simulink model "open loop simulationHbridgeMLI"  (R2019a)
settings: Solver=VariableStepAuto  StartTime=0.0  StopTime=0.2  RelTol=1e-3
libraries: powerlib x73, simulink x13, powerlib_meascontrol x3
settings Model: Creator=BPW  LastModifiedBy=BPW

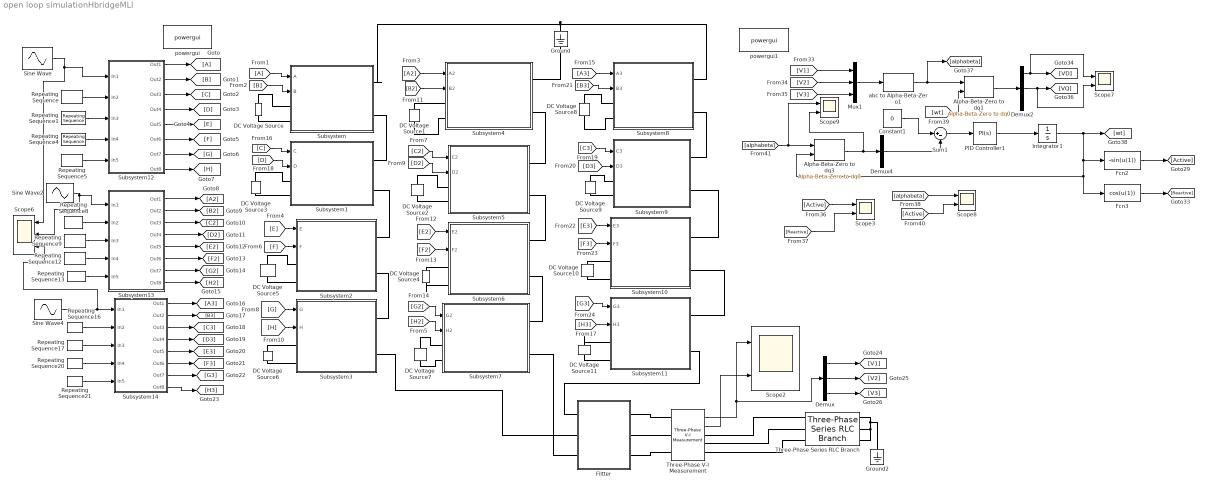
== system open loop simulationHbridgeMLI ==
  Alpha-Beta-Zero to dq1 : powerlib_meascontrol/Transformations/Alpha-Beta-Zero to dq0  Alignment=90 degrees behind phase A axis
      settings: SourceProductName=Simscape Electrical
  Alpha-Beta-Zero to dq3 : powerlib_meascontrol/Transformations/Alpha-Beta-Zero to dq0  Alignment=90 degrees behind phase A axis
      settings: SourceProductName=Simscape Electrical
  Constant1 : Constant  Value=0
  DC Voltage Source{,1..11} (12 alike) : powerlib/Electrical Sources/DC Voltage Source  Amplitude=-100  Measurements=None
      settings: SourceProductName=Simscape Electrical
  Demux : Demux  Outputs=3
  Demux2 : Demux  Outputs=3
  Demux4 : Demux  Outputs=3
  Fcn2 : Fcn  Expr=-sin(u(1))
  Fcn3 : Fcn  Expr=cos(u(1))
  Filtter : Subsystem
  Ground : powerlib/Elements/Ground  LConnTagsString=a
      settings: SourceProductName=Simscape Electrical
  Ground2 : powerlib/Elements/Ground  LConnTagsString=a
      settings: SourceProductName=Simscape Electrical
  Integrator1 : Integrator
  Mux1 : Mux  Inputs=3
  PID Controller1 : simulink/Continuous/PID Controller  Controller=PI  Form=Parallel  TimeDomain=Continuous-time  SampleTime=-1  IntegratorMethod=Forward Euler  FilterMethod=Forward Euler  ControllerParametersSource=internal  P=1  I=170  D=0  UseFilter=on  N=100  TunerSelectOption=Transfer Function Based (PID Tuner App)  InitialConditionSource=internal  InitialConditionForIntegrator=0  InitialConditionForFilter=0  DifferentiatorICPrevScaledInput=0  ExternalReset=none  TrackingMode=off  Kt=1  LimitOutput=off  UpperSaturationLimit=inf  LowerSaturationLimit=-inf  LinearizeAsGain=on  AntiWindupMode=none  Kb=1  POutMin=[]  POutMax=[]  IOutMin=[]  IOutMax=[]  DOutMin=[]  DOutMax=[]  NOutMin=[]  NOutMax=[]  SumOutMin=[]  SumOutMax=[]  SaturationOutMin=[]  SaturationOutMax=[]  PParamMin=[]  PParamMax=[]  IParamMin=[]  IParamMax=[]  DParamMin=[]  DParamMax=[]  NParamMin=[]  NParamMax=[]  KbParamMin=[]  KbParamMax=[]  KtParamMin=[]  KtParamMax=[]  KbOutMin=[]  KbOutMax=[]  KtOutMin=[]  KtOutMax=[]  IntegratorOutMin=[]  IntegratorOutMax=[]  FilterOutMin=[]  FilterOutMax=[]  SumI1OutMin=[]  SumI1OutMax=[]  SumI2OutMin=[]  SumI2OutMax=[]  SumI3OutMin=[]  SumI3OutMax=[]  SumI4OutMin=[]  SumI4OutMax=[]  SumDOutMin=[]  SumDOutMax=[]  DifferentiatorOutMin=[]  DifferentiatorOutMax=[]  FilterDiffOutCoefMin=[]  FilterDiffOutCoefMax=[]  ReciprocalOutMin=[]  ReciprocalOutMax=[]  SumDenOutMin=[]  SumDenOutMax=[]  SumNumOutMin=[]  SumNumOutMax=[]  DivideOutMin=[]  DivideOutMax=[]  IntegratorContinuousStateAttributes=''  IntegratorStateMustResolveToSignalObject=off  IntegratorRTWStateStorageClass=Auto  FilterContinuousStateAttributes=''  FilterStateMustResolveToSignalObject=off  FilterRTWStateStorageClass=Auto  ParallelPVariant=InternalParameters  IdealPVariant=Disabled  IVariant=InternalParameters  DVariant=Disabled  IntegratorVariant=Continuous  SatVariant=Disabled  AWVariant=Passthrough  PCopyVariant=Disabled  TRVariant=Disabled  FdbkBlocksVariant=Forward  IdealPFdbkVariant=Disabled  SatFdbkVariant=Disabled  DerivativeFilterVariant=Disabled  NVariant=Disabled  NCopyVariant=Disabled_SignalSpec  FilterICVariant=Disabled  IntegratorICVariant=InternalICs  ExternalResetVariant=Disabled  TRSumVariant=Passthrough  SumFdbkVariant=Disabled  SumVariant=Sum_PI
  Repeating Sequence : simulink/Sources/Repeating Sequence  rep_seq_t=[0 1e-4]  rep_seq_y=[0 1]
  Repeating Sequence1 : simulink/Sources/Repeating Sequence  rep_seq_t=[0 1e-4]  rep_seq_y=[1 2]
  Repeating Sequence12 : simulink/Sources/Repeating Sequence  rep_seq_t=[0 1e-4]  rep_seq_y=[2 3]
  Repeating Sequence13 : simulink/Sources/Repeating Sequence  rep_seq_t=[0 1e-4]  rep_seq_y=[3 4]
  Repeating Sequence16 : simulink/Sources/Repeating Sequence  rep_seq_t=[0 1e-4]  rep_seq_y=[0 1]
  Repeating Sequence17 : simulink/Sources/Repeating Sequence  rep_seq_t=[0 1e-4]  rep_seq_y=[1 2]
  Repeating Sequence20 : simulink/Sources/Repeating Sequence  rep_seq_t=[0 1e-4]  rep_seq_y=[2 3]
  Repeating Sequence21 : simulink/Sources/Repeating Sequence  rep_seq_t=[0 1e-4]  rep_seq_y=[3 4]
  Repeating Sequence4 : simulink/Sources/Repeating Sequence  rep_seq_t=[0 1e-4]  rep_seq_y=[2 3]
  Repeating Sequence5 : simulink/Sources/Repeating Sequence  rep_seq_t=[0 1e-4]  rep_seq_y=[3 4]
  Repeating Sequence8 : simulink/Sources/Repeating Sequence  rep_seq_t=[0 1e-4]  rep_seq_y=[0 1]
  Repeating Sequence9 : simulink/Sources/Repeating Sequence  rep_seq_t=[0 1e-4]  rep_seq_y=[1 2]
  Scope{2..3,7..9} (5 alike) : Scope  NumInputPorts=2
  Scope6 : Scope  NumInputPorts=3
  Sine Wave : Sin  Amplitude=4  Frequency=314.15  SampleTime=0
  Sine Wave2 : Sin  Amplitude=4  Frequency=314.15  Phase=2*pi/3  SampleTime=0
  Sine Wave4 : Sin  Amplitude=4  Frequency=314.15  Phase=4*pi/3  SampleTime=0
  Subsystem : Subsystem
  Subsystem1 : Subsystem
  Subsystem10 : Subsystem
  Subsystem11 : Subsystem
  Subsystem12 : Subsystem
  Subsystem13 : Subsystem
  Subsystem14 : Subsystem
  Subsystem2 : Subsystem
  Subsystem3 : Subsystem
  Subsystem4 : Subsystem
  Subsystem5 : Subsystem
  Subsystem6 : Subsystem
  Subsystem7 : Subsystem
  Subsystem8 : Subsystem
  Subsystem9 : Subsystem
  Sum1 : Sum  Inputs=|+-
  Three-Phase Series RLC Branch : powerlib/Elements/Three-Phase Series RLC Branch  LConnTagsString=A|B|C  RConnTagsString=A|B|C  BranchType=R  Resistance=10  Inductance=1e-9  Capacitance=1e-6  Measurements=None
      settings: SourceProductName=Simscape Electrical
  Three-Phase V-I Measurement : powerlib/Measurements/Three-Phase V-I Measurement  VoltageMeasurement=phase-to-ground  SetLabelV=off  LabelV=Vabc  Vpu=off  VpuLL=off  CurrentMeasurement=yes  SetLabelI=off  LabelI=Iabc  Ipu=off  Pbase=100e6  Vbase=500e3  OutputType=Complex  PhasorSimulation=off  PSBequivalent=0
      settings: SourceProductName=Simscape Electrical
  abc to Alpha-Beta-Zero1 : powerlib_meascontrol/Transformations/abc to Alpha-Beta-Zero
      settings: SourceProductName=Simscape Electrical
  powergui : powerlib/powergui  Priority=1  SimulationMode=Discrete  SampleTime=5e-5  frequency=60  Iterations=50  frequencyindice=0  Pbase=100e6  ErrMax=1e-4  UnitsV=kV  UnitsW=MW  buscounter=0  FunctionMessages=off  echomessages=off  EnableUseOfTLC=off  CurrentSourceSwitches=off  DisableSnubberDevices=off  DisableRonSwitches=off  DisableVfSwitches=off  DisplayEquations=off  AutomaticDiscreteSolvers=off  SolverType=Tustin/Backward Euler (TBE)  Interpol=off  ExternalGateDelay=off  methode=off  Ts=100  x0status=blocks  SPID=on  SwTol=0  HookPort=off  NonlinearTolerance=0  nMaxIteration=15  ContinueOnMaxIteration=off  RestoreLinks=warning  ResistiveCurrentMeasurement=off  Frange=[0:2:500]  Ylog=off  Xlog=on  ShowGrid=off  save=off  variable=ZData  structure=0  ZoomFFT=off  StartTime=0.0  cycles=1  DisplayStyle=1  fundamental=60  FreqAxis=off  MaxFrequency=1000  frequencyindicesteady=1  RmsSteady=1  display=off
      settings: SourceProductName=Simscape Electrical
  powergui1 : powerlib/powergui  Priority=1  SimulationMode=Discrete  SampleTime=5e-5  frequency=60  Iterations=50  frequencyindice=0  Pbase=100e6  ErrMax=1e-4  UnitsV=kV  UnitsW=MW  buscounter=0  FunctionMessages=off  echomessages=off  EnableUseOfTLC=off  CurrentSourceSwitches=off  DisableSnubberDevices=off  DisableRonSwitches=off  DisableVfSwitches=off  DisplayEquations=off  AutomaticDiscreteSolvers=off  SolverType=Tustin/Backward Euler (TBE)  Interpol=off  ExternalGateDelay=off  methode=off  Ts=100  x0status=blocks  SPID=on  SwTol=0  HookPort=off  NonlinearTolerance=0  nMaxIteration=15  ContinueOnMaxIteration=off  RestoreLinks=warning  ResistiveCurrentMeasurement=off  Frange=[0:2:500]  Ylog=off  Xlog=on  ShowGrid=off  save=off  variable=ZData  structure=0  ZoomFFT=off  StartTime=0.0  cycles=1  DisplayStyle=1  fundamental=60  FreqAxis=off  MaxFrequency=1000  frequencyindicesteady=1  RmsSteady=1  display=off
      settings: SourceProductName=Simscape Electrical
  wires:
  [B3] -> Subsystem8/2("B3 ")
  [A3] -> Subsystem8/1(A3)
  [F3] -> Subsystem10/2(F3)
  [C3] -> Subsystem9/1("C3 ")
  [E3] -> Subsystem10/1(E3)
  [H2] -> Subsystem7/2("H2 ")
  [B2] -> Subsystem4/2("B2 ")
  [G2] -> Subsystem7/1(G2)
  [C] -> Subsystem1/1(C)
  [H3] -> Subsystem11/2("H3 ")
  [E2] -> Subsystem6/1(E2)
  [F] -> Subsystem2/2(F)
  [A] -> Subsystem/1(A)
  [C2] -> Subsystem5/1(C2)
  [F2] -> Subsystem6/2(F2)
  [D] -> Subsystem1/2("D ")
  [D3] -> Subsystem9/2("D3 ")
  [B] -> Subsystem/2(B)
  [H] -> Subsystem3/2("H ")
  [G] -> Subsystem3/1(G)
  [A2] -> Subsystem4/1("A2 ")
  [G3] -> Subsystem11/1(G3)
  [E] -> Subsystem2/1(E)
  [D2] -> Subsystem5/2("D2 ")
  Three-Phase V-I Measurement/2 -> Scope2/2
  Demux/1 -> [V1]
  Demux/3 -> [V3]
  Demux/2 -> [V2]
  Three-Phase V-I Measurement/1 -> Scope2/1, Demux/1
  Subsystem12/7(Out7) -> [G]
  Subsystem12/4(Out4) -> [D]
  Subsystem12/6(Out6) -> [F]
  Subsystem14/3(Out3) -> [C3]
  Repeating Sequence20/1 -> Subsystem14/4(In4)
  Subsystem14/6(Out6) -> [F3]
  Subsystem12/2(Out2) -> [B]
  Repeating Sequence/1 -> Subsystem12/2(In2)
  Repeating Sequence1/1 -> Subsystem12/3(In3)
  Subsystem12/3(Out3) -> [C]
  Subsystem12/8(Out8) -> [H]
  Subsystem12/5(Out5) -> [E]
  Subsystem13/7(Out7) -> [G2]
  Subsystem13/6(Out6) -> [F2]
  Subsystem13/8(Out8) -> [H2]
  Subsystem12/1(Out1) -> [A]
  Subsystem13/4(Out4) -> [D2]
  Subsystem13/2(Out2) -> [B2]
  Subsystem13/1(Out1) -> [A2]
  Subsystem14/7(Out7) -> [G3]
  Repeating Sequence21/1 -> Subsystem14/5(In5)
  Repeating Sequence5/1 -> Subsystem12/5(In5)
  Repeating Sequence8/1 -> Subsystem13/2(In2)
  Subsystem14/8(Out8) -> [H3]
  Repeating Sequence17/1 -> Subsystem14/3(In3)
  Sine Wave2/1 -> Scope6/2, Subsystem13/1(In1)
  Repeating Sequence13/1 -> Subsystem13/5(In5)
  Repeating Sequence16/1 -> Subsystem14/2(In2)
  Subsystem14/1(Out1) -> [A3]
  Subsystem14/2(Out2) -> [B3]
  Sine Wave4/1 -> Scope6/3, Subsystem14/1(In1)
  Subsystem14/4(Out4) -> [D3]
  Subsystem13/5(Out5) -> [E2]
  Subsystem14/5(Out5) -> [E3]
  Repeating Sequence4/1 -> Subsystem12/4(In4)
  Sine Wave/1 -> Scope6/1, Subsystem12/1(In1)
  Subsystem13/3(Out3) -> [C2]
  Repeating Sequence12/1 -> Subsystem13/4(In4)
  Repeating Sequence9/1 -> Subsystem13/3(In3)
  [alphabeta] -> Scope8/1
  Demux4/2 -> Sum1/2
  Demux2/1 -> [VD], Scope7/1
  Alpha-Beta-Zero to dq1/1 -> Demux2/1
  Fcn3/1 -> [Reactive]
  [Active] -> Scope3/1
  Integrator1/1 -> Fcn2/1, Fcn3/1, Alpha-Beta-Zero to dq3/2, [wt]
  Demux2/2 -> Scope7/2, [VQ]
  [Reactive] -> Scope3/2
  [Active] -> Scope8/2
  Fcn2/1 -> [Active]
  Mux1/1 -> abc to Alpha-Beta-Zero1/1
  [V1] -> Mux1/1
  [wt] -> Alpha-Beta-Zero to dq1/2
  abc to Alpha-Beta-Zero1/1 -> Alpha-Beta-Zero to dq1/1, [alphabeta]
  Constant1/1 -> Sum1/1
  [V3] -> Mux1/3
  [alphabeta] -> Scope9/1, Alpha-Beta-Zero to dq3/1
  PID Controller1/1 -> Integrator1/1
  Alpha-Beta-Zero to dq3/1 -> Scope9/2, Demux4/1
  Sum1/1 -> PID Controller1/1
  [V2] -> Mux1/2
  connections:
  Ground/LConn1 -- Subsystem/RConn1 -- Subsystem4/RConn1 -- Subsystem8/RConn1
  Subsystem3/LConn1 -- DC Voltage Source6/RConn1
  Subsystem8/LConn1 -- DC Voltage Source8/RConn1
  Subsystem8/LConn2 -- DC Voltage Source8/LConn1
  Subsystem11/LConn2 -- DC Voltage Source11/LConn1
  Subsystem2/LConn1 -- DC Voltage Source5/RConn1
  Subsystem2/LConn2 -- DC Voltage Source5/LConn1
  Subsystem10/RConn2 -- Subsystem11/RConn1
  Subsystem10/RConn1 -- Subsystem9/RConn2
  Subsystem10/LConn1 -- DC Voltage Source10/RConn1
  Subsystem4/LConn1 -- DC Voltage Source1/RConn1
  Subsystem5/LConn2 -- DC Voltage Source2/LConn1
  Subsystem2/RConn1 -- Subsystem1/RConn2
  Subsystem5/LConn1 -- DC Voltage Source2/RConn1
  Subsystem7/LConn2 -- DC Voltage Source7/LConn1
  Subsystem6/RConn1 -- Subsystem5/RConn2
  Subsystem4/RConn2 -- Subsystem5/RConn1
  Subsystem6/LConn1 -- DC Voltage Source4/RConn1
  Subsystem8/RConn2 -- Subsystem9/RConn1
  Subsystem9/LConn1 -- DC Voltage Source9/RConn1
  Subsystem2/RConn2 -- Subsystem3/RConn1
  Subsystem9/LConn2 -- DC Voltage Source9/LConn1
  Subsystem3/LConn2 -- DC Voltage Source6/LConn1
  Subsystem4/LConn2 -- DC Voltage Source1/LConn1
  Subsystem6/RConn2 -- Subsystem7/RConn1
  Subsystem/RConn2 -- Subsystem1/RConn1
  Subsystem10/LConn2 -- DC Voltage Source10/LConn1
  Subsystem/LConn2 -- DC Voltage Source/LConn1
  Subsystem1/LConn1 -- DC Voltage Source3/RConn1
  Three-Phase Series RLC Branch/LConn1 -- Ground2/LConn1 -- Three-Phase Series RLC Branch/LConn3 -- Three-Phase Series RLC Branch/LConn2
  Three-Phase Series RLC Branch/RConn1 -- Three-Phase V-I Measurement/RConn1
  Three-Phase V-I Measurement/RConn2 -- Three-Phase Series RLC Branch/RConn2
  Three-Phase V-I Measurement/RConn3 -- Three-Phase Series RLC Branch/RConn3
  DC Voltage Source4/LConn1 -- Subsystem6/LConn2
  DC Voltage Source11/RConn1 -- Subsystem11/LConn1
  DC Voltage Source7/RConn1 -- Subsystem7/LConn1
  Subsystem/LConn1 -- DC Voltage Source/RConn1
  Subsystem1/LConn2 -- DC Voltage Source3/LConn1
  Subsystem11/RConn2 -- Filtter/LConn1
  Filtter/LConn2 -- Subsystem3/RConn2
  Filtter/LConn3 -- Subsystem7/RConn2
  Three-Phase V-I Measurement/LConn1 -- Filtter/RConn1
  Three-Phase V-I Measurement/LConn2 -- Filtter/RConn2
  Three-Phase V-I Measurement/LConn3 -- Filtter/RConn3

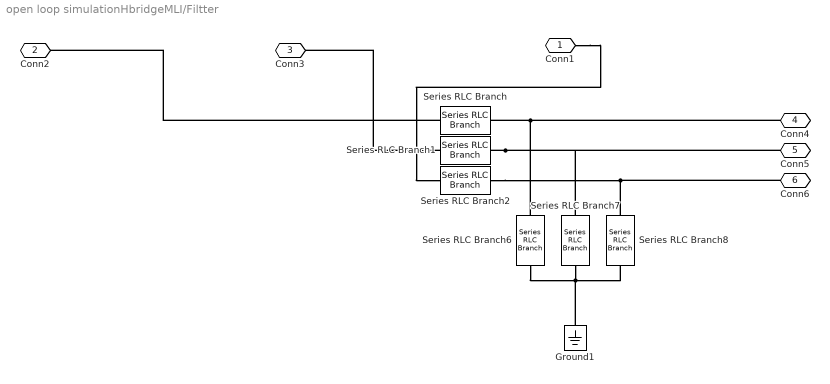
== system open loop simulationHbridgeMLI/Filtter ==
  Ground1 : powerlib/Elements/Ground  LConnTagsString=a
      settings: SourceProductName=Simscape Electrical
  Series RLC Branch : powerlib/Elements/Series RLC Branch  LConnTagsString=__new0  RConnTagsString=__new0  BranchType=L  Resistance=1  Inductance=500e-6  SetiL0=off  InitialCurrent=0  Capacitance=1e-6  Setx0=off  InitialVoltage=0  Measurements=None
      settings: SourceProductName=Simscape Electrical
  Series RLC Branch1 : powerlib/Elements/Series RLC Branch  LConnTagsString=__new0  RConnTagsString=__new0  BranchType=L  Resistance=1  Inductance=500e-6  SetiL0=off  InitialCurrent=0  Capacitance=1e-6  Setx0=off  InitialVoltage=0  Measurements=None
      settings: SourceProductName=Simscape Electrical
  Series RLC Branch2 : powerlib/Elements/Series RLC Branch  LConnTagsString=__new0  RConnTagsString=__new0  BranchType=L  Resistance=1  Inductance=500e-6  SetiL0=off  InitialCurrent=0  Capacitance=1e-6  Setx0=off  InitialVoltage=0  Measurements=None
      settings: SourceProductName=Simscape Electrical
  Series RLC Branch6 : powerlib/Elements/Series RLC Branch  LConnTagsString=__new0  RConnTagsString=__new0  BranchType=C  Resistance=1  Inductance=500e-6  SetiL0=off  InitialCurrent=0  Capacitance=1000e-6  Setx0=off  InitialVoltage=0  Measurements=None
      settings: SourceProductName=Simscape Electrical
  Series RLC Branch7 : powerlib/Elements/Series RLC Branch  LConnTagsString=__new0  RConnTagsString=__new0  BranchType=C  Resistance=1  Inductance=500e-6  SetiL0=off  InitialCurrent=0  Capacitance=1000e-6  Setx0=off  InitialVoltage=0  Measurements=None
      settings: SourceProductName=Simscape Electrical
  Series RLC Branch8 : powerlib/Elements/Series RLC Branch  LConnTagsString=__new0  RConnTagsString=__new0  BranchType=C  Resistance=1  Inductance=500e-6  SetiL0=off  InitialCurrent=0  Capacitance=1000e-6  Setx0=off  InitialVoltage=0  Measurements=None
      settings: SourceProductName=Simscape Electrical
  Conn1 : PMIOPort  Side=Left
  Conn2 : PMIOPort  Port=2  Side=Left
  Conn3 : PMIOPort  Port=3  Side=Left
  Conn4 : PMIOPort  Port=4  Side=Right
  Conn5 : PMIOPort  Port=5  Side=Right
  Conn6 : PMIOPort  Port=6  Side=Right
  connections:
  Series RLC Branch7/RConn1 -- Ground1/LConn1 -- Series RLC Branch8/RConn1 -- Series RLC Branch6/RConn1
  Series RLC Branch1/RConn1 -- Conn5/RConn1 -- Series RLC Branch7/LConn1
  Series RLC Branch8/LConn1 -- Conn6/RConn1 -- Series RLC Branch2/RConn1
  Series RLC Branch6/LConn1 -- Conn4/RConn1 -- Series RLC Branch/RConn1
  Series RLC Branch/LConn1 -- Conn2/RConn1
  Conn1/RConn1 -- Series RLC Branch2/LConn1
  Series RLC Branch1/LConn1 -- Conn3/RConn1

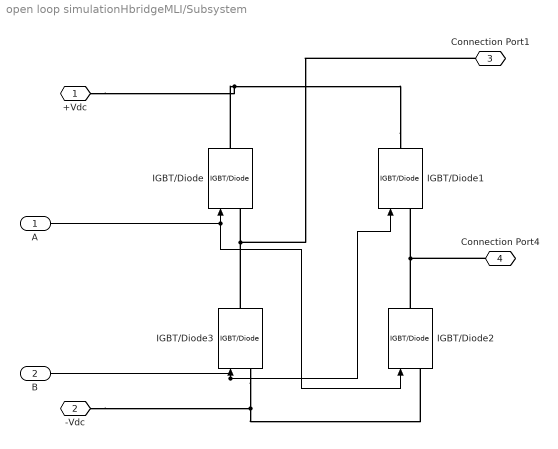
== system open loop simulationHbridgeMLI/Subsystem ==
  A : Inport
  B : Inport  Port=2
  IGBT/Diode{,1..3} (4 alike) : powerlib/Power Electronics/IGBT//Diode  Ron=1e-3  Rs=1e5  Cs=inf  Measurements=off
      settings: SourceProductName=Simscape Electrical
  +Vdc : PMIOPort  Side=Left
  -Vdc : PMIOPort  Port=2  Side=Left
  Connection Port1 : PMIOPort  Port=3  Side=Right
  Connection Port4 : PMIOPort  Port=4  Side=Right
  wires:
  A/1 -> IGBT/Diode2/1, IGBT/Diode/1
  B/1 -> IGBT/Diode1/1, IGBT/Diode3/1
  connections:
  IGBT/Diode3/RConn1 -- IGBT/Diode/LConn1 -- Connection Port1/RConn1
  IGBT/Diode1/RConn1 -- IGBT/Diode/RConn1 -- +Vdc/RConn1
  IGBT/Diode1/LConn1 -- IGBT/Diode2/RConn1 -- Connection Port4/RConn1
  IGBT/Diode2/LConn1 -- IGBT/Diode3/LConn1 -- -Vdc/RConn1

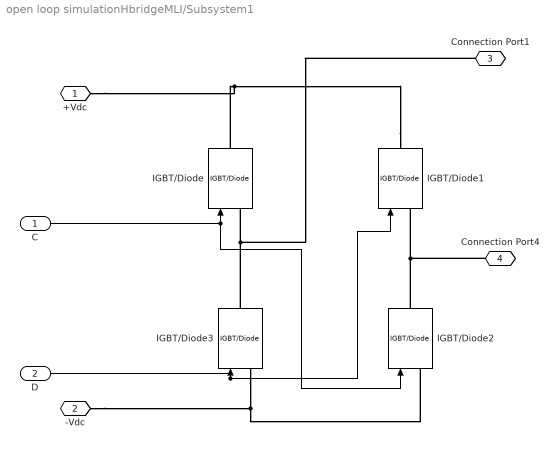
== system open loop simulationHbridgeMLI/Subsystem1 ==
  C : Inport
  "D " : Inport  Port=2
  IGBT/Diode{,1..3} (4 alike) : powerlib/Power Electronics/IGBT//Diode  Ron=1e-3  Rs=1e5  Cs=inf  Measurements=off
      settings: SourceProductName=Simscape Electrical
  +Vdc : PMIOPort  Side=Left
  -Vdc : PMIOPort  Port=2  Side=Left
  Connection Port1 : PMIOPort  Port=3  Side=Right
  Connection Port4 : PMIOPort  Port=4  Side=Right
  wires:
  C/1 -> IGBT/Diode2/1, IGBT/Diode/1
  "D "/1 -> IGBT/Diode1/1, IGBT/Diode3/1
  connections:
  IGBT/Diode3/RConn1 -- IGBT/Diode/LConn1 -- Connection Port1/RConn1
  IGBT/Diode1/RConn1 -- IGBT/Diode/RConn1 -- +Vdc/RConn1
  IGBT/Diode1/LConn1 -- IGBT/Diode2/RConn1 -- Connection Port4/RConn1
  IGBT/Diode2/LConn1 -- IGBT/Diode3/LConn1 -- -Vdc/RConn1

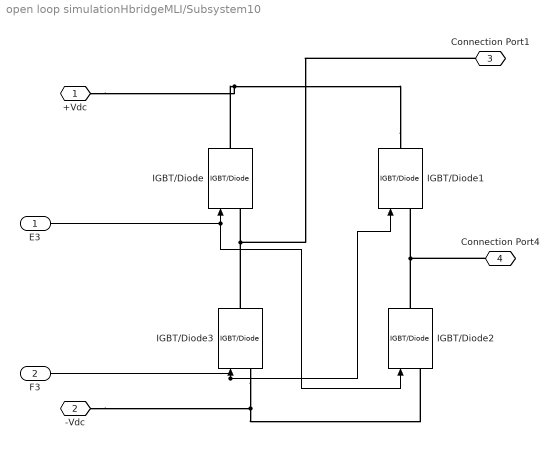
== system open loop simulationHbridgeMLI/Subsystem10 ==
  E3 : Inport
  F3 : Inport  Port=2
  IGBT/Diode{,1..3} (4 alike) : powerlib/Power Electronics/IGBT//Diode  Ron=1e-3  Rs=1e5  Cs=inf  Measurements=off
      settings: SourceProductName=Simscape Electrical
  +Vdc : PMIOPort  Side=Left
  -Vdc : PMIOPort  Port=2  Side=Left
  Connection Port1 : PMIOPort  Port=3  Side=Right
  Connection Port4 : PMIOPort  Port=4  Side=Right
  wires:
  E3/1 -> IGBT/Diode2/1, IGBT/Diode/1
  F3/1 -> IGBT/Diode1/1, IGBT/Diode3/1
  connections:
  IGBT/Diode3/RConn1 -- IGBT/Diode/LConn1 -- Connection Port1/RConn1
  IGBT/Diode1/RConn1 -- IGBT/Diode/RConn1 -- +Vdc/RConn1
  IGBT/Diode1/LConn1 -- IGBT/Diode2/RConn1 -- Connection Port4/RConn1
  IGBT/Diode2/LConn1 -- IGBT/Diode3/LConn1 -- -Vdc/RConn1

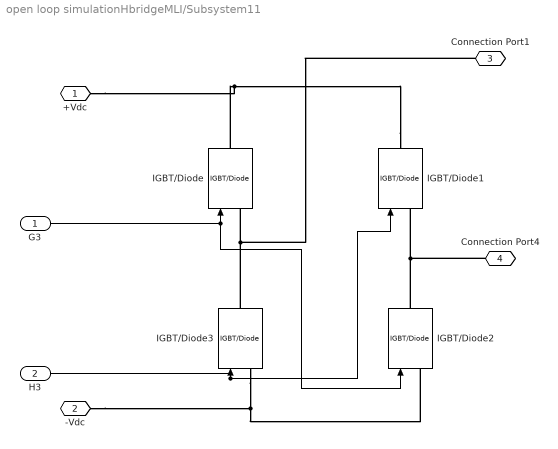
== system open loop simulationHbridgeMLI/Subsystem11 ==
  G3 : Inport
  "H3 " : Inport  Port=2
  IGBT/Diode{,1..3} (4 alike) : powerlib/Power Electronics/IGBT//Diode  Ron=1e-3  Rs=1e5  Cs=inf  Measurements=off
      settings: SourceProductName=Simscape Electrical
  +Vdc : PMIOPort  Side=Left
  -Vdc : PMIOPort  Port=2  Side=Left
  Connection Port1 : PMIOPort  Port=3  Side=Right
  Connection Port4 : PMIOPort  Port=4  Side=Right
  wires:
  G3/1 -> IGBT/Diode2/1, IGBT/Diode/1
  "H3 "/1 -> IGBT/Diode1/1, IGBT/Diode3/1
  connections:
  IGBT/Diode3/RConn1 -- IGBT/Diode/LConn1 -- Connection Port1/RConn1
  IGBT/Diode1/RConn1 -- IGBT/Diode/RConn1 -- +Vdc/RConn1
  IGBT/Diode1/LConn1 -- IGBT/Diode2/RConn1 -- Connection Port4/RConn1
  IGBT/Diode2/LConn1 -- IGBT/Diode3/LConn1 -- -Vdc/RConn1

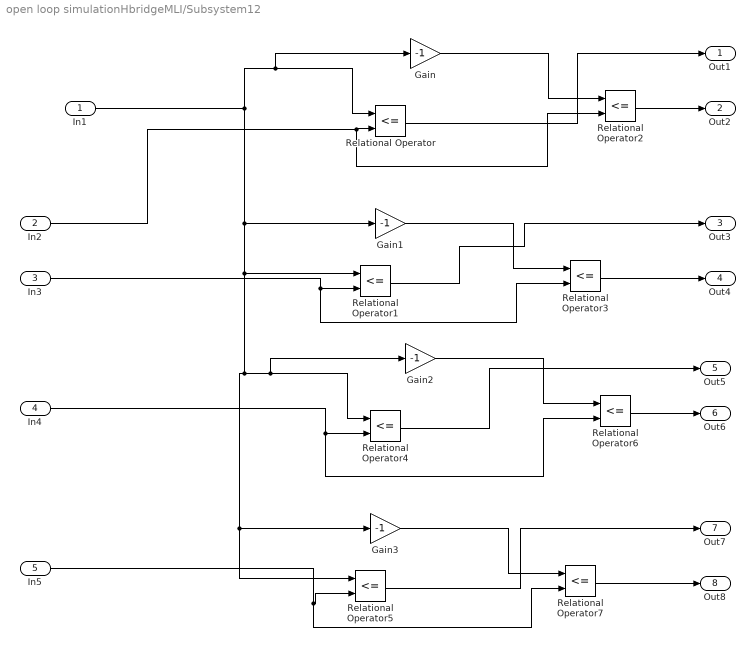
== system open loop simulationHbridgeMLI/Subsystem12 ==
  In1 : Inport
  In2 : Inport  Port=2
  In3 : Inport  Port=3
  In4 : Inport  Port=4
  In5 : Inport  Port=5
  Gain{,1..3} (4 alike) : Gain  Gain=-1
  Relational Operator{,1..7} (8 alike) : RelationalOperator  Operator=<=  OutDataTypeStr=boolean  RndMeth=Simplest
  Out1 : Outport
  Out2 : Outport  Port=2
  Out3 : Outport  Port=3
  Out4 : Outport  Port=4
  Out5 : Outport  Port=5
  Out6 : Outport  Port=6
  Out7 : Outport  Port=7
  Out8 : Outport  Port=8
  wires:
  In5/1 -> Relational Operator7/2, Relational Operator5/2
  In2/1 -> Relational Operator/2, Relational Operator2/2
  In1/1 -> Gain3/1, Relational Operator5/1, Gain2/1, Relational Operator4/1, Relational Operator1/1, Gain1/1, Gain/1, Relational Operator/1
  Gain/1 -> Relational Operator2/1
  In4/1 -> Relational Operator6/2, Relational Operator4/2
  In3/1 -> Relational Operator3/2, Relational Operator1/2
  Relational Operator4/1 -> Out5/1
  Gain2/1 -> Relational Operator6/1
  Relational Operator3/1 -> Out4/1
  Gain3/1 -> Relational Operator7/1
  Gain1/1 -> Relational Operator3/1
  Relational Operator/1 -> Out1/1
  Relational Operator2/1 -> Out2/1
  Relational Operator7/1 -> Out8/1
  Relational Operator6/1 -> Out6/1
  Relational Operator1/1 -> Out3/1
  Relational Operator5/1 -> Out7/1

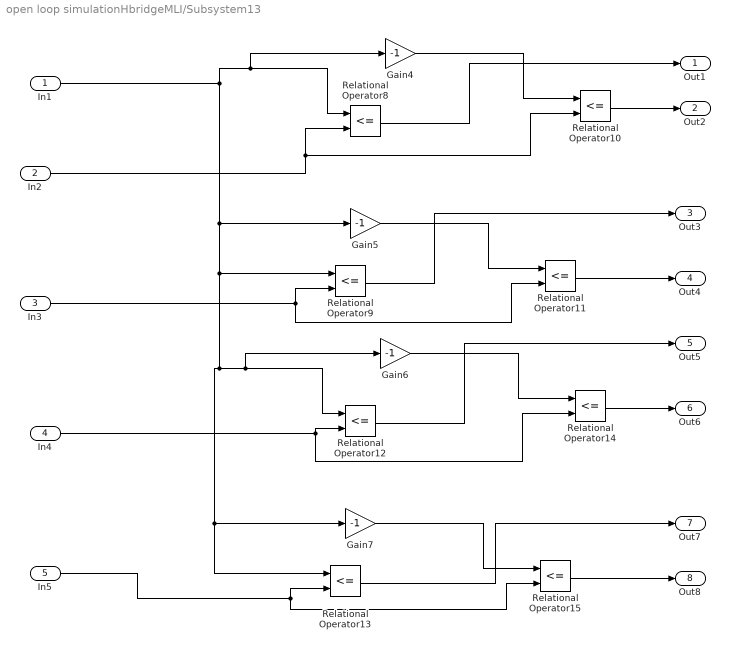
== system open loop simulationHbridgeMLI/Subsystem13 ==
  In1 : Inport
  In2 : Inport  Port=2
  In3 : Inport  Port=3
  In4 : Inport  Port=4
  In5 : Inport  Port=5
  Gain{4..7} (4 alike) : Gain  Gain=-1
  Relational Operator{8..15} (8 alike) : RelationalOperator  Operator=<=  OutDataTypeStr=boolean  RndMeth=Simplest
  Out1 : Outport
  Out2 : Outport  Port=2
  Out3 : Outport  Port=3
  Out4 : Outport  Port=4
  Out5 : Outport  Port=5
  Out6 : Outport  Port=6
  Out7 : Outport  Port=7
  Out8 : Outport  Port=8
  wires:
  In2/1 -> Relational Operator8/2, Relational Operator10/2
  In1/1 -> Gain7/1, Relational Operator13/1, Gain6/1, Relational Operator12/1, Relational Operator9/1, Gain5/1, Gain4/1, Relational Operator8/1
  Gain6/1 -> Relational Operator14/1
  Gain7/1 -> Relational Operator15/1
  In4/1 -> Relational Operator12/2, Relational Operator14/2
  In3/1 -> Relational Operator9/2, Relational Operator11/2
  Gain5/1 -> Relational Operator11/1
  Gain4/1 -> Relational Operator10/1
  In5/1 -> Relational Operator15/2, Relational Operator13/2
  Relational Operator11/1 -> Out4/1
  Relational Operator14/1 -> Out6/1
  Relational Operator15/1 -> Out8/1
  Relational Operator10/1 -> Out2/1
  Relational Operator8/1 -> Out1/1
  Relational Operator9/1 -> Out3/1
  Relational Operator13/1 -> Out7/1
  Relational Operator12/1 -> Out5/1

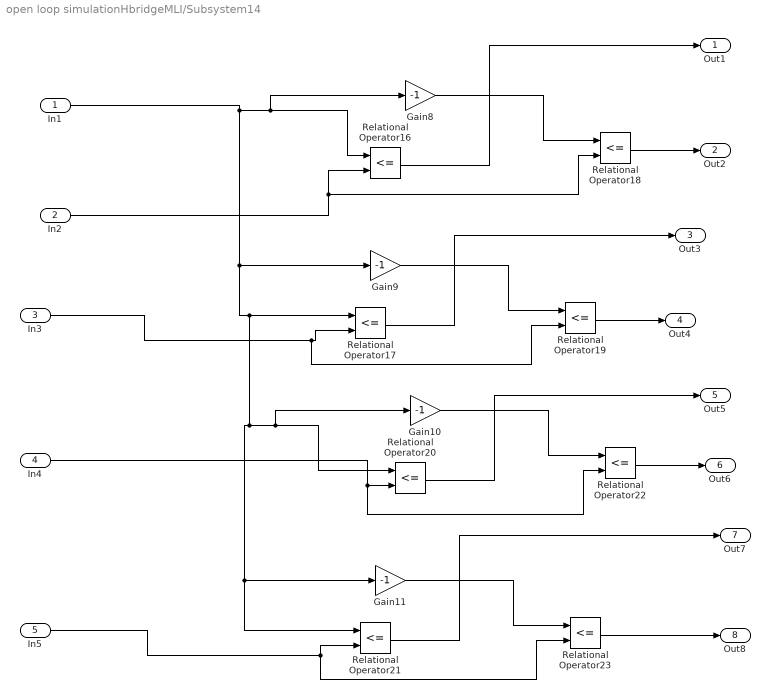
== system open loop simulationHbridgeMLI/Subsystem14 ==
  In1 : Inport
  In2 : Inport  Port=2
  In3 : Inport  Port=3
  In4 : Inport  Port=4
  In5 : Inport  Port=5
  Gain{8..11} (4 alike) : Gain  Gain=-1
  Relational Operator{16..23} (8 alike) : RelationalOperator  Operator=<=  OutDataTypeStr=boolean  RndMeth=Simplest
  Out1 : Outport
  Out2 : Outport  Port=2
  Out3 : Outport  Port=3
  Out4 : Outport  Port=4
  Out5 : Outport  Port=5
  Out6 : Outport  Port=6
  Out7 : Outport  Port=7
  Out8 : Outport  Port=8
  wires:
  In3/1 -> Relational Operator19/2, Relational Operator17/2
  In4/1 -> Relational Operator22/2, Relational Operator20/2
  In5/1 -> Relational Operator23/2, Relational Operator21/2
  In2/1 -> Relational Operator16/2, Relational Operator18/2
  Gain9/1 -> Relational Operator19/1
  In1/1 -> Gain9/1, Gain11/1, Relational Operator21/1, Gain10/1, Relational Operator20/1, Relational Operator17/1, Gain8/1, Relational Operator16/1
  Gain8/1 -> Relational Operator18/1
  Gain11/1 -> Relational Operator23/1
  Gain10/1 -> Relational Operator22/1
  Relational Operator17/1 -> Out3/1
  Relational Operator21/1 -> Out7/1
  Relational Operator22/1 -> Out6/1
  Relational Operator23/1 -> Out8/1
  Relational Operator16/1 -> Out1/1
  Relational Operator19/1 -> Out4/1
  Relational Operator18/1 -> Out2/1
  Relational Operator20/1 -> Out5/1

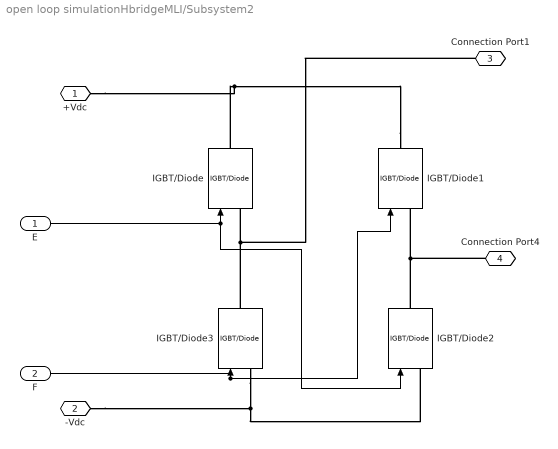
== system open loop simulationHbridgeMLI/Subsystem2 ==
  E : Inport
  F : Inport  Port=2
  IGBT/Diode{,1..3} (4 alike) : powerlib/Power Electronics/IGBT//Diode  Ron=1e-3  Rs=1e5  Cs=inf  Measurements=off
      settings: SourceProductName=Simscape Electrical
  +Vdc : PMIOPort  Side=Left
  -Vdc : PMIOPort  Port=2  Side=Left
  Connection Port1 : PMIOPort  Port=3  Side=Right
  Connection Port4 : PMIOPort  Port=4  Side=Right
  wires:
  E/1 -> IGBT/Diode2/1, IGBT/Diode/1
  F/1 -> IGBT/Diode1/1, IGBT/Diode3/1
  connections:
  IGBT/Diode3/RConn1 -- IGBT/Diode/LConn1 -- Connection Port1/RConn1
  IGBT/Diode1/RConn1 -- IGBT/Diode/RConn1 -- +Vdc/RConn1
  IGBT/Diode1/LConn1 -- IGBT/Diode2/RConn1 -- Connection Port4/RConn1
  IGBT/Diode2/LConn1 -- IGBT/Diode3/LConn1 -- -Vdc/RConn1

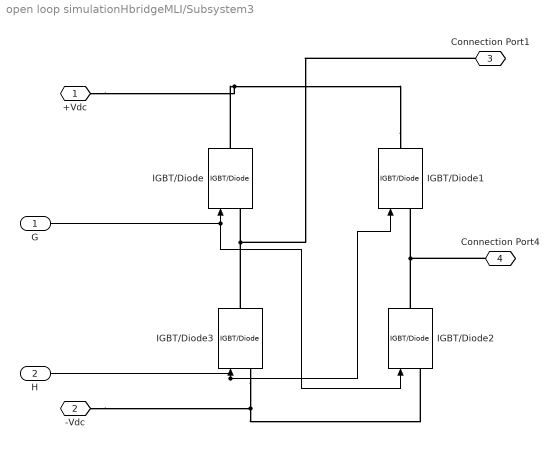
== system open loop simulationHbridgeMLI/Subsystem3 ==
  G : Inport
  "H " : Inport  Port=2
  IGBT/Diode{,1..3} (4 alike) : powerlib/Power Electronics/IGBT//Diode  Ron=1e-3  Rs=1e5  Cs=inf  Measurements=off
      settings: SourceProductName=Simscape Electrical
  +Vdc : PMIOPort  Side=Left
  -Vdc : PMIOPort  Port=2  Side=Left
  Connection Port1 : PMIOPort  Port=3  Side=Right
  Connection Port4 : PMIOPort  Port=4  Side=Right
  wires:
  G/1 -> IGBT/Diode2/1, IGBT/Diode/1
  "H "/1 -> IGBT/Diode1/1, IGBT/Diode3/1
  connections:
  IGBT/Diode3/RConn1 -- IGBT/Diode/LConn1 -- Connection Port1/RConn1
  IGBT/Diode1/RConn1 -- IGBT/Diode/RConn1 -- +Vdc/RConn1
  IGBT/Diode1/LConn1 -- IGBT/Diode2/RConn1 -- Connection Port4/RConn1
  IGBT/Diode2/LConn1 -- IGBT/Diode3/LConn1 -- -Vdc/RConn1

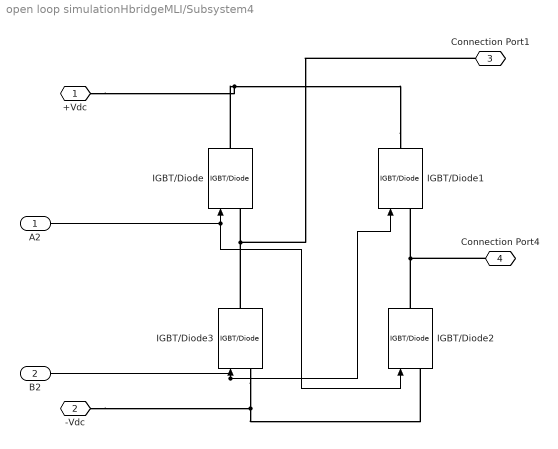
== system open loop simulationHbridgeMLI/Subsystem4 ==
  "A2 " : Inport
  "B2 " : Inport  Port=2
  IGBT/Diode{,1..3} (4 alike) : powerlib/Power Electronics/IGBT//Diode  Ron=1e-3  Rs=1e5  Cs=inf  Measurements=off
      settings: SourceProductName=Simscape Electrical
  +Vdc : PMIOPort  Side=Left
  -Vdc : PMIOPort  Port=2  Side=Left
  Connection Port1 : PMIOPort  Port=3  Side=Right
  Connection Port4 : PMIOPort  Port=4  Side=Right
  wires:
  "A2 "/1 -> IGBT/Diode2/1, IGBT/Diode/1
  "B2 "/1 -> IGBT/Diode1/1, IGBT/Diode3/1
  connections:
  IGBT/Diode3/RConn1 -- IGBT/Diode/LConn1 -- Connection Port1/RConn1
  IGBT/Diode1/RConn1 -- IGBT/Diode/RConn1 -- +Vdc/RConn1
  IGBT/Diode1/LConn1 -- IGBT/Diode2/RConn1 -- Connection Port4/RConn1
  IGBT/Diode2/LConn1 -- IGBT/Diode3/LConn1 -- -Vdc/RConn1

== system open loop simulationHbridgeMLI/Subsystem5 ==
  C2 : Inport
  "D2 " : Inport  Port=2
  IGBT/Diode{,1..3} (4 alike) : powerlib/Power Electronics/IGBT//Diode  Ron=1e-3  Rs=1e5  Cs=inf  Measurements=off
      settings: SourceProductName=Simscape Electrical
  +Vdc : PMIOPort  Side=Left
  -Vdc : PMIOPort  Port=2  Side=Left
  Connection Port1 : PMIOPort  Port=3  Side=Right
  Connection Port4 : PMIOPort  Port=4  Side=Right
  wires:
  C2/1 -> IGBT/Diode2/1, IGBT/Diode/1
  "D2 "/1 -> IGBT/Diode1/1, IGBT/Diode3/1
  connections:
  IGBT/Diode3/RConn1 -- IGBT/Diode/LConn1 -- Connection Port1/RConn1
  IGBT/Diode1/RConn1 -- IGBT/Diode/RConn1 -- +Vdc/RConn1
  IGBT/Diode1/LConn1 -- IGBT/Diode2/RConn1 -- Connection Port4/RConn1
  IGBT/Diode2/LConn1 -- IGBT/Diode3/LConn1 -- -Vdc/RConn1

== system open loop simulationHbridgeMLI/Subsystem6 ==
  E2 : Inport
  F2 : Inport  Port=2
  IGBT/Diode{,1..3} (4 alike) : powerlib/Power Electronics/IGBT//Diode  Ron=1e-3  Rs=1e5  Cs=inf  Measurements=off
      settings: SourceProductName=Simscape Electrical
  +Vdc : PMIOPort  Side=Left
  -Vdc : PMIOPort  Port=2  Side=Left
  Connection Port1 : PMIOPort  Port=3  Side=Right
  Connection Port4 : PMIOPort  Port=4  Side=Right
  wires:
  E2/1 -> IGBT/Diode2/1, IGBT/Diode/1
  F2/1 -> IGBT/Diode1/1, IGBT/Diode3/1
  connections:
  IGBT/Diode3/RConn1 -- IGBT/Diode/LConn1 -- Connection Port1/RConn1
  IGBT/Diode1/RConn1 -- IGBT/Diode/RConn1 -- +Vdc/RConn1
  IGBT/Diode1/LConn1 -- IGBT/Diode2/RConn1 -- Connection Port4/RConn1
  IGBT/Diode2/LConn1 -- IGBT/Diode3/LConn1 -- -Vdc/RConn1

== system open loop simulationHbridgeMLI/Subsystem7 ==
  G2 : Inport
  "H2 " : Inport  Port=2
  IGBT/Diode{,1..3} (4 alike) : powerlib/Power Electronics/IGBT//Diode  Ron=1e-3  Rs=1e5  Cs=inf  Measurements=off
      settings: SourceProductName=Simscape Electrical
  +Vdc : PMIOPort  Side=Left
  -Vdc : PMIOPort  Port=2  Side=Left
  Connection Port1 : PMIOPort  Port=3  Side=Right
  Connection Port4 : PMIOPort  Port=4  Side=Right
  wires:
  G2/1 -> IGBT/Diode2/1, IGBT/Diode/1
  "H2 "/1 -> IGBT/Diode1/1, IGBT/Diode3/1
  connections:
  IGBT/Diode3/RConn1 -- IGBT/Diode/LConn1 -- Connection Port1/RConn1
  IGBT/Diode1/RConn1 -- IGBT/Diode/RConn1 -- +Vdc/RConn1
  IGBT/Diode1/LConn1 -- IGBT/Diode2/RConn1 -- Connection Port4/RConn1
  IGBT/Diode2/LConn1 -- IGBT/Diode3/LConn1 -- -Vdc/RConn1

== system open loop simulationHbridgeMLI/Subsystem8 ==
  A3 : Inport
  "B3 " : Inport  Port=2
  IGBT/Diode{,1..3} (4 alike) : powerlib/Power Electronics/IGBT//Diode  Ron=1e-3  Rs=1e5  Cs=inf  Measurements=off
      settings: SourceProductName=Simscape Electrical
  +Vdc : PMIOPort  Side=Left
  -Vdc : PMIOPort  Port=2  Side=Left
  Connection Port1 : PMIOPort  Port=3  Side=Right
  Connection Port4 : PMIOPort  Port=4  Side=Right
  wires:
  A3/1 -> IGBT/Diode2/1, IGBT/Diode/1
  "B3 "/1 -> IGBT/Diode1/1, IGBT/Diode3/1
  connections:
  IGBT/Diode3/RConn1 -- IGBT/Diode/LConn1 -- Connection Port1/RConn1
  IGBT/Diode1/RConn1 -- IGBT/Diode/RConn1 -- +Vdc/RConn1
  IGBT/Diode1/LConn1 -- IGBT/Diode2/RConn1 -- Connection Port4/RConn1
  IGBT/Diode2/LConn1 -- IGBT/Diode3/LConn1 -- -Vdc/RConn1

== system open loop simulationHbridgeMLI/Subsystem9 ==
  "C3 " : Inport
  "D3 " : Inport  Port=2
  IGBT/Diode{,1..3} (4 alike) : powerlib/Power Electronics/IGBT//Diode  Ron=1e-3  Rs=1e5  Cs=inf  Measurements=off
      settings: SourceProductName=Simscape Electrical
  +Vdc : PMIOPort  Side=Left
  -Vdc : PMIOPort  Port=2  Side=Left
  Connection Port1 : PMIOPort  Port=3  Side=Right
  Connection Port4 : PMIOPort  Port=4  Side=Right
  wires:
  "C3 "/1 -> IGBT/Diode2/1, IGBT/Diode/1
  "D3 "/1 -> IGBT/Diode1/1, IGBT/Diode3/1
  connections:
  IGBT/Diode3/RConn1 -- IGBT/Diode/LConn1 -- Connection Port1/RConn1
  IGBT/Diode1/RConn1 -- IGBT/Diode/RConn1 -- +Vdc/RConn1
  IGBT/Diode1/LConn1 -- IGBT/Diode2/RConn1 -- Connection Port4/RConn1
  IGBT/Diode2/LConn1 -- IGBT/Diode3/LConn1 -- -Vdc/RConn1
